simulink model "SignalProcessing2"  (R2023a)
settings: Solver=VariableStepAuto  StartTime=0.0  StopTime=191  RelTol=1e-3
settings Model: Creator=mohsen.amiri  LastModifiedBy=mohsen.amiri

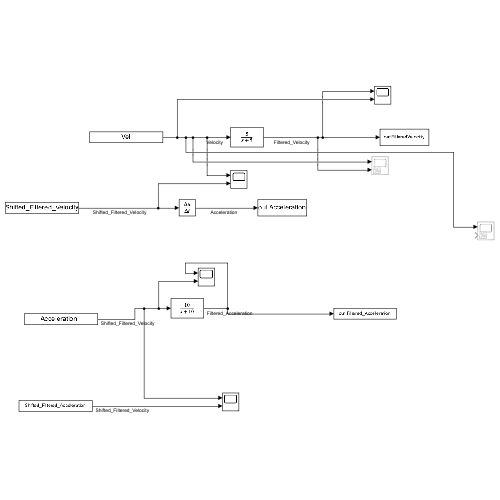
[thumbnail: Simulink's stored preview of the top-level diagram]
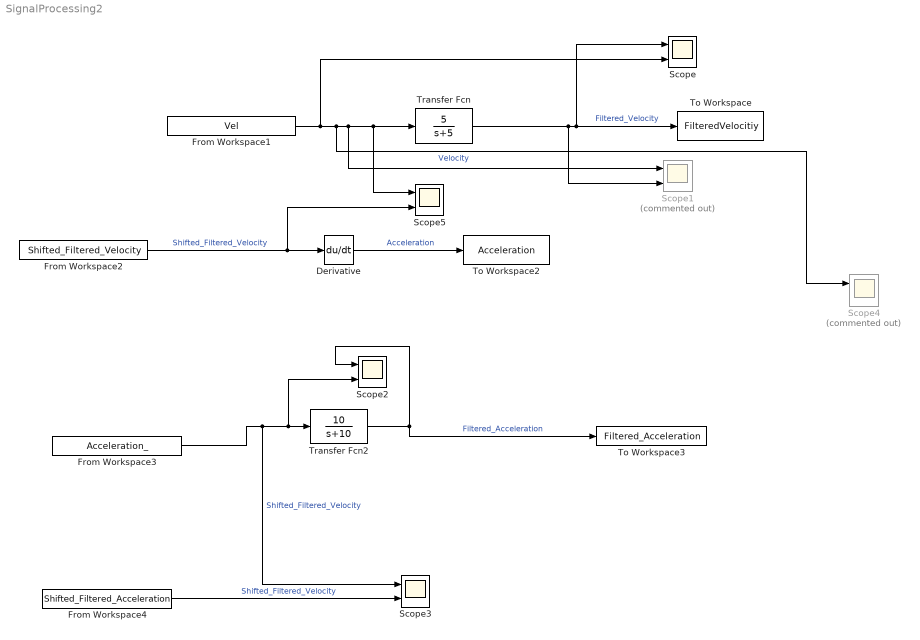
== system SignalProcessing2 ==
  Derivative : Derivative
  From Workspace1 : FromWorkspace  VariableName=Vel  OutDataTypeStr=double  SampleTime=0.008333333333212
  From Workspace2 : FromWorkspace  VariableName=Shifted_Filtered_Velocity  OutDataTypeStr=double  SampleTime=0.008333333333212
  From Workspace3 : FromWorkspace  VariableName=Acceleration_  OutDataTypeStr=double  SampleTime=0.008333333333212
  From Workspace4 : FromWorkspace  VariableName=Shifted_Filtered_Acceleration  OutDataTypeStr=double  SampleTime=0.008333333333212
  Scope{,2..3,5} (4 alike) : Scope  NumInputPorts=2
  Scope1 : Scope  Commented=on  NumInputPorts=2
  Scope4 : Scope  Commented=on  NumInputPorts=2
  To Workspace : ToWorkspace  VariableName=FilteredVelocitiy  SampleTime=0.008333333333212
  To Workspace2 : ToWorkspace  VariableName=Acceleration  SampleTime=0.008333333333212
  To Workspace3 : ToWorkspace  VariableName=Filtered_Acceleration  SampleTime=0.008333333333212
  Transfer Fcn : TransferFcn  Numerator=[5]  Denominator=[1 5]
  Transfer Fcn2 : TransferFcn  Numerator=[10]  Denominator=[1 10]
  wires:
  From Workspace2/1 -> Scope5/2, Derivative/1  "Shifted_Filtered_Velocity"
  Derivative/1 -> To Workspace2/1  "Acceleration"
  From Workspace1/1 -> Scope/2, Scope4/1, Scope1/1, Scope5/1, Transfer Fcn/1  "Velocity"
  Transfer Fcn/1 -> Scope1/2, Scope/1, To Workspace/1  "Filtered_Velocity"
  From Workspace3/1 -> Scope3/1, Scope2/2, Transfer Fcn2/1  "Shifted_Filtered_Velocity"
  Transfer Fcn2/1 -> Scope2/1, To Workspace3/1  "Filtered_Acceleration"
  From Workspace4/1 -> Scope3/2  "Shifted_Filtered_Velocity"
